simulink model "untitled"  (R2017b)
settings: Solver=VariableStepAuto  StartTime=0.0  StopTime=10.0  RelTol=1e-3
settings Model: Creator=Administrator  LastModifiedBy=Administrator

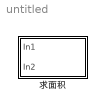
== system untitled ==
  求面积 : Subsystem

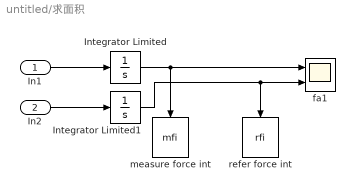
== system untitled/求面积 ==
  In1 : Inport
  In2 : Inport  Port=2
  Integrator Limited : Integrator  UpperSaturationLimit=1  LowerSaturationLimit=0  ZeroCross=off
  Integrator Limited1 : Integrator  UpperSaturationLimit=1  LowerSaturationLimit=0  ZeroCross=off
  fa1 : Scope  NumInputPorts=2
  measure force int : ToWorkspace  VariableName=mfi  SaveFormat=Timeseries  SampleTime=-1
  refer force int : ToWorkspace  VariableName=rfi  SaveFormat=Timeseries  SampleTime=-1
  wires:
  Integrator Limited1/1 -> refer force int/1, fa1/2
  Integrator Limited/1 -> fa1/1, measure force int/1
  In2/1 -> Integrator Limited1/1
  In1/1 -> Integrator Limited/1
